simulink library "send_to_unity"  (Simulink 9.0)
settings: Solver=VariableStepAuto  StartTime=0.0  StopTime=10.0  RelTol=1e-3  EnableMultiTasking=on
undefined symbols (not defined in the file): localhost
libraries: simunity x2, instrumentlib x1
settings Model: SuppressorTable=22 serialization::archive 11 0 6 0 0 0 0 0  Creator=tinglihu  LastModifiedBy=johannes

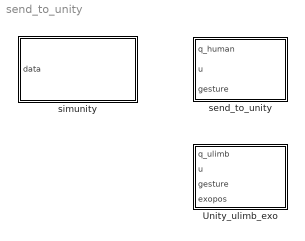
== system send_to_unity ==
  Unity_ulimb_exo : Subsystem
  send_to_unity : Subsystem  mask{ip='localhost', port=8051}
      mask prompts: ip "Remote address (ip)"; port "Port (port)"
      mask help:
      | Sends data to Unity using udp.
      |
      | Input:
      | q_human [1x12]
      | u [1x42]
      | gesture [1x2]
  simunity : Subsystem  mask{ip=localhost, port=8051}
      mask prompts: ip "Remote address (ip)"; port "Port (port)"
      mask Display: image('unity.png')

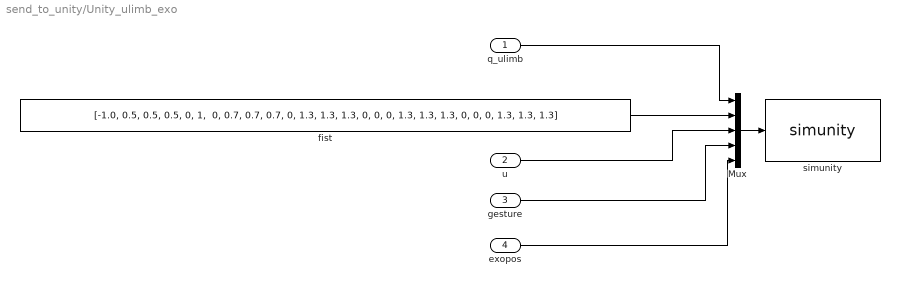
== system send_to_unity/Unity_ulimb_exo ==
  q_ulimb : Inport
  u : Inport  Port=2
  gesture : Inport  Port=3
  exopos : Inport  Port=4
  Mux : Mux  Inputs=[12, 26, 42, 2 15]
  fist : Constant  Value="[-1.0, 0.5, 0.5, 0.5, 0, 1,  0, 0.7, 0.7, 0.7, 0, 1.3, 1.3, 1.3, 0, 0, 0, 1.3, 1.3, 1.3, 0, 0, 0, 1.3, 1.3, 1.3]"
  simunity : simunity/simunity  SystemSampleTime=-1
  wires:
  fist/1 -> Mux/2
  q_ulimb/1 -> Mux/1
  Mux/1 -> simunity/1
  gesture/1 -> Mux/4
  u/1 -> Mux/3
  exopos/1 -> Mux/5

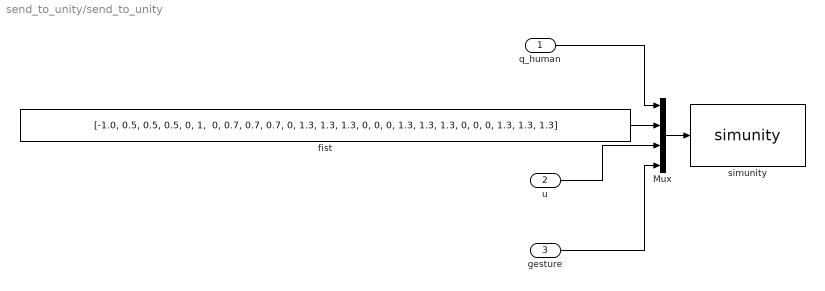
== system send_to_unity/send_to_unity ==
  q_human : Inport
  u : Inport  Port=2
  gesture : Inport  Port=3
  Mux : Mux  Inputs=[12, 26, 42, 2]
  fist : Constant  Value="[-1.0, 0.5, 0.5, 0.5, 0, 1,  0, 0.7, 0.7, 0.7, 0, 1.3, 1.3, 1.3, 0, 0, 0, 1.3, 1.3, 1.3, 0, 0, 0, 1.3, 1.3, 1.3]"
  simunity : simunity/simunity  SystemSampleTime=-1
  wires:
  fist/1 -> Mux/2
  q_human/1 -> Mux/1
  Mux/1 -> simunity/1
  gesture/1 -> Mux/4
  u/1 -> Mux/3

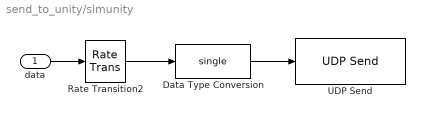
== system send_to_unity/simunity ==
  data : Inport
  Data Type Conversion : DataTypeConversion  OutDataTypeStr=single  RndMeth=Round
  Rate Transition2 : RateTransition  OutPortSampleTime=1/50
  UDP Send : instrumentlib/UDP Send  Host=localhost  Port=8051  LocalPort=-1  EnableBlockingMode=on  ByteOrder=LittleEndian
      settings: SourceProductName=Instrument Control Toolbox
  wires:
  Rate Transition2/1 -> Data Type Conversion/1
  data/1 -> Rate Transition2/1
  Data Type Conversion/1 -> UDP Send/1
